simulink model "DPT_model_practice_3"  (R2021b)
settings: Solver=FixedStepAuto  StartTime=0.0  StopTime=0.5  FixedStep=1e-3  RelTol=1e-3
values from neighbouring files (symbols this model uses):
  Jn = 2*Jd    (= 0.000334)    [practice_3_script.m]
  Kd = place(SYS.A,SYS.B,p)    [practice_3_script.m]
  ke = (Un-R*In)/wn    (= 0.320333333333)    [practice_3_script.m]
  km = Mn/In    (= 0.228971962617)    [practice_3_script.m]
  ku = 20    [practice_3_script.m]
  L = l'    [practice_3_script.m]
  La = 10^-3 * 58    (= 0.058)    [practice_3_script.m]
  R = 8.5    [practice_3_script.m]
  SYS = ss(Ad,Bd,Cd,Dd)    [practice_3_script.m]
settings Model: Creator=vkad  LastModifiedBy=vkad

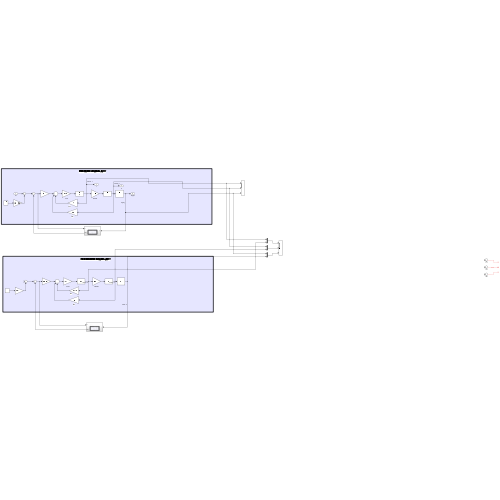
[thumbnail: Simulink's stored preview of the top-level diagram]
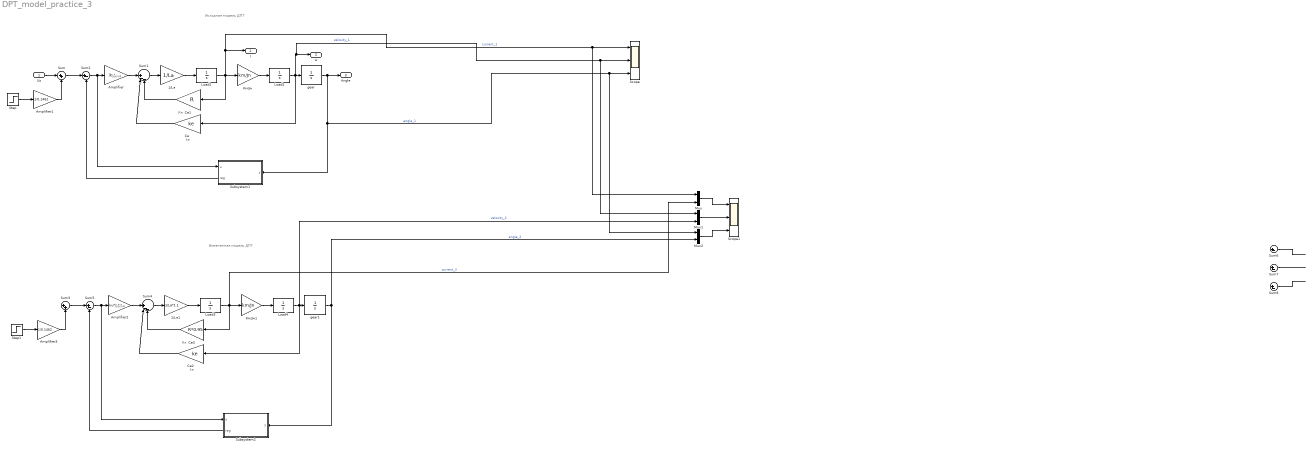
== system DPT_model_practice_3 ==
  note: Rя
  note: Исходная модель ДПТ
  note: Gain4
  note: kе
  note: Rя
  note: Измененная модель ДПТ
  note: Gain4
  note: kе
  Uz : Inport
  1/Lя : Gain  Gain=1/La
  1/Lя1 : Gain  Gain=1/La*1.1
  Amplifier : Gain  Gain=ku
  Amplifier1 : Gain  Gain=1/0.1462
  Amplifier2 : Gain  Gain=ku*0.95
  Amplifier3 : Gain  Gain=1/0.1462
  Ce : Gain  Gain=ke
  Ce1 : Gain  Gain=R
  Ce2 : Gain  Gain=ke
  Ce3 : Gain  Gain=R*0.95
  Load{1..4} (4 alike) : TransferFcn  Denominator=[1 0]
  Mux : Mux  Inputs=2
  Mux1 : Mux  Inputs=2
  Mux2 : Mux  Inputs=2
  Scope : Scope  NumInputPorts=3
  Scope1 : Scope  NumInputPorts=3
  Step : Step  Time=0  SampleTime=0
  Step1 : Step  Time=0  SampleTime=0
  Subsystem1 : Subsystem
      settings: PortSchema="{\"entries\":[{\"content\":{\"sides\":[{\"content\":{\"connectorIds\":[\"In1\",\"Out1\"]},\"type\":\"ConnectorPlacement.EquallySpacedRectSide\",\"uuid\":\"1ae5a343-437d-4cb9-9822-e2db9fa7010c\"},{\"content\":{\"connectorIds\":[\"In2\"],\"side\":\"RIGHT\"},\"type\":\"ConnectorPlacement.EquallySpacedRectSide\",\"uuid\":\"a13fd255-885b-49a4-bdfe-42517e7d2bb6\"},{\"content\":{\"connectorIds\":[],\"side\":\"TOP\"},\"type\":\"ConnectorPlacement.EquallySpacedRectSide\",\"uuid\":\"ec77d7e4-a70f-42b2-8285-e16af54c9a8e\"}]},\"type\":\"ConnectorPlacement.EquallySpacedConnector\",\"uuid\":\"a53451af-0313-4fad-91e1-dbe8374f8c5a\"}],\"packageUris\":[\"http://schema.mathworks.com/mf0/Connector/R2020b\"],\"version\":\"1.0\"}"
  Subsystem2 : Subsystem
      settings: PortSchema="{\"entries\":[{\"content\":{\"sides\":[{\"content\":{\"connectorIds\":[\"In1\",\"Out1\"]},\"type\":\"ConnectorPlacement.EquallySpacedRectSide\",\"uuid\":\"1ae5a343-437d-4cb9-9822-e2db9fa7010c\"},{\"content\":{\"connectorIds\":[\"In2\"],\"side\":\"RIGHT\"},\"type\":\"ConnectorPlacement.EquallySpacedRectSide\",\"uuid\":\"a13fd255-885b-49a4-bdfe-42517e7d2bb6\"},{\"content\":{\"connectorIds\":[],\"side\":\"TOP\"},\"type\":\"ConnectorPlacement.EquallySpacedRectSide\",\"uuid\":\"ec77d7e4-a70f-42b2-8285-e16af54c9a8e\"}]},\"type\":\"ConnectorPlacement.EquallySpacedConnector\",\"uuid\":\"a53451af-0313-4fad-91e1-dbe8374f8c5a\"}],\"packageUris\":[\"http://schema.mathworks.com/mf0/Connector/R2020b\"],\"version\":\"1.0\"}"
  Sum : Sum  Inputs=|++
  Sum1 : Sum  Inputs=||+--
  Sum{2,5..8} (5 alike) : Sum  Inputs=|+-
  Sum3 : Sum  Inputs=|++
  Sum4 : Sum  Inputs=||+--
  gear : TransferFcn  Numerator=1  Denominator=[1 0]
  gear1 : TransferFcn  Numerator=1  Denominator=[1 0]
  Км/Jн : Gain  Gain=km/Jn
  Км/Jн1 : Gain  Gain=km/Jn
  I : Outport
  w : Outport  Port=2
  Angle : Outport  Port=3
  wires:
  Км/Jн/1 -> Load2/1
  Ce/1 -> Sum1/2
  Sum/1 -> Sum2/1
  1/Lя/1 -> Load1/1
  Sum2/1 -> Subsystem1/1(u), Amplifier/1
  Uz/1 -> Sum/1
  Ce1/1 -> Sum1/3
  gear/1 -> Subsystem1/2(y), Mux2/1, Scope/3, Angle/1  "angle_1"
  Step/1 -> Amplifier1/1
  Amplifier/1 -> Sum1/1
  Sum1/1 -> 1/Lя/1
  Load2/1 -> Mux1/1, Scope/2, w/1, Ce/1, gear/1  "velosity_1"
  Load1/1 -> Ce1/1, Км/Jн/1, Mux/1, Scope/1, I/1  "current_1"
  Amplifier1/1 -> Sum/2
  Amplifier3/1 -> Sum3/2
  Subsystem2/1(reg) -> Sum5/2
  Load3/1 -> Mux/2, Км/Jн1/1, Ce3/1  "current_2"
  Load4/1 -> Mux1/2, gear1/1, Ce2/1  "velosity_2"
  Sum4/1 -> 1/Lя1/1
  Amplifier2/1 -> Sum4/1
  Step1/1 -> Amplifier3/1
  gear1/1 -> Mux2/2, Subsystem2/2(y)  "angle_2"
  Ce3/1 -> Sum4/3
  Sum5/1 -> Subsystem2/1(u), Amplifier2/1
  1/Lя1/1 -> Load3/1
  Sum3/1 -> Sum5/1
  Ce2/1 -> Sum4/2
  Км/Jн1/1 -> Load4/1
  Subsystem1/1(reg) -> Sum2/2
  Mux1/1 -> Scope1/2
  Mux2/1 -> Scope1/3
  Mux/1 -> Scope1/1
  Sum8/1 -> ?
  Sum7/1 -> ?
  Sum6/1 -> ?

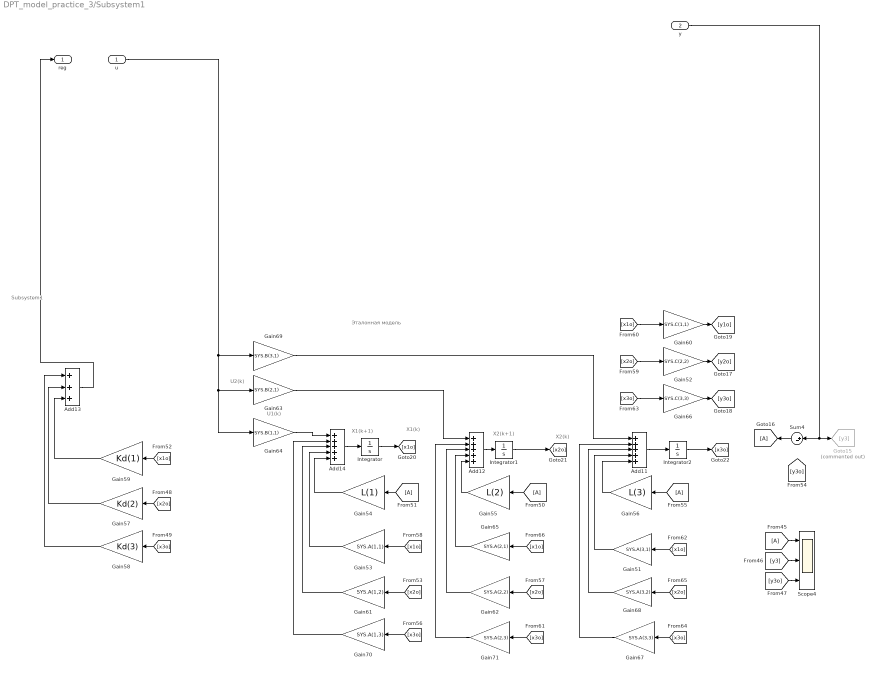
== system DPT_model_practice_3/Subsystem1 ==
  note: Subsystem1
  note: U2(k)
  note: U1(k)
  note: X2(k+1)
  note: X1(k+1)
  note: X2(k)
  note: X1(k)
  note: Эталонная модель
  u : Inport
  y : Inport  Port=2
  Add11 : Sum  Inputs=+++++
  Add12 : Sum  Inputs=+++++
  Add13 : Sum  Inputs=+++
  Add14 : Sum  Inputs=+++++
  Gain51 : Gain  Gain=SYS.A(3,1)
  Gain52 : Gain  Gain=SYS.C(2,2)
  Gain53 : Gain  Gain=SYS.A(1,1)
  Gain54 : Gain  Gain=L(1)
  Gain55 : Gain  Gain=L(2)
  Gain56 : Gain  Gain=L(3)
  Gain57 : Gain  Gain=Kd(2)
  Gain58 : Gain  Gain=Kd(3)
  Gain59 : Gain  Gain=Kd(1)
  Gain60 : Gain  Gain=SYS.C(1,1)
  Gain61 : Gain  Gain=SYS.A(1,2)
  Gain62 : Gain  Gain=SYS.A(2,2)
  Gain63 : Gain  Gain=SYS.B(2,1)
  Gain64 : Gain  Gain=SYS.B(1,1)
  Gain65 : Gain  Gain=SYS.A(2,1)
  Gain66 : Gain  Gain=SYS.C(3,3)
  Gain67 : Gain  Gain=SYS.A(3,3)
  Gain68 : Gain  Gain=SYS.A(3,2)
  Gain69 : Gain  Gain=SYS.B(3,1)
  Gain70 : Gain  Gain=SYS.A(1,3)
  Gain71 : Gain  Gain=SYS.A(2,3)
  Goto15 : Goto  Commented=on  GotoTag=y3
  Integrator : Integrator
  Integrator1 : Integrator
  Integrator2 : Integrator
  Scope4 : Scope  NumInputPorts=3
  Sum4 : Sum  Inputs=|+-
  reg : Outport
  wires:
  u/1 -> Gain69/1, Gain64/1, Gain63/1
  [x1o] -> Gain65/1
  Gain53/1 -> Add14/4
  [y3] -> Scope4/2
  Gain69/1 -> Add11/1
  [A] -> Scope4/1
  [x2o] -> Gain68/1
  Gain61/1 -> Add14/3
  Gain63/1 -> Add12/1
  Gain60/1 -> [y1o]
  [y3o] -> Scope4/3
  [x3o] -> Gain70/1
  [x2o] -> Gain61/1
  Gain58/1 -> Add13/1
  Gain67/1 -> Add11/2
  [A] -> Gain55/1
  Gain54/1 -> Add14/5
  Sum4/1 -> [A]
  y/1 -> Sum4/1, Goto15/1
  [x1o] -> Gain51/1
  Gain59/1 -> Add13/3
  [x3o] -> Gain67/1
  [x1o] -> Gain59/1
  Gain70/1 -> Add14/2
  Gain55/1 -> Add12/5
  [x2o] -> Gain62/1
  [x2o] -> Gain57/1
  [x1o] -> Gain53/1
  [A] -> Gain56/1
  [x1o] -> Gain60/1
  Gain51/1 -> Add11/4
  Gain52/1 -> [y2o]
  Gain71/1 -> Add12/2
  [A] -> Gain54/1
  [x2o] -> Gain52/1
  Gain56/1 -> Add11/5
  Gain62/1 -> Add12/3
  Gain68/1 -> Add11/3
  [x3o] -> Gain71/1
  [x3o] -> Gain58/1
  Gain66/1 -> [y3o]
  Gain64/1 -> Add14/1
  Gain65/1 -> Add12/4
  Gain57/1 -> Add13/2
  [x3o] -> Gain66/1
  Add13/1 -> reg/1
  Add14/1 -> Integrator/1
  Integrator/1 -> [x1o]
  Add12/1 -> Integrator1/1
  Integrator1/1 -> [x2o]
  Add11/1 -> Integrator2/1
  Integrator2/1 -> [x3o]

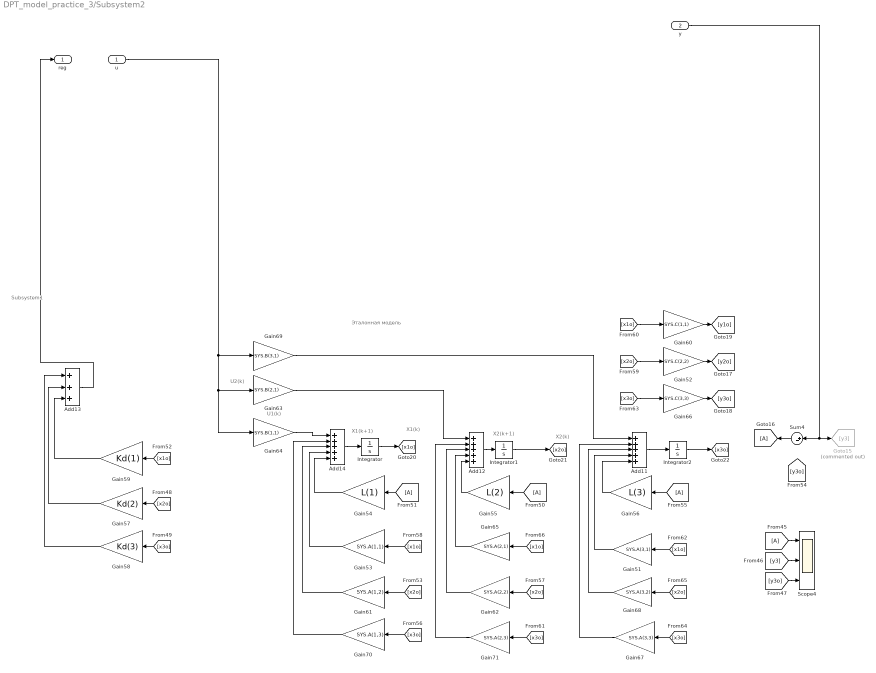
== system DPT_model_practice_3/Subsystem2 ==
  note: Эталонная модель
  note: X1(k)
  note: X2(k)
  note: X1(k+1)
  note: X2(k+1)
  note: U1(k)
  note: U2(k)
  note: Subsystem1
  u : Inport
  y : Inport  Port=2
  Add11 : Sum  Inputs=+++++
  Add12 : Sum  Inputs=+++++
  Add13 : Sum  Inputs=+++
  Add14 : Sum  Inputs=+++++
  Gain51 : Gain  Gain=SYS.A(3,1)
  Gain52 : Gain  Gain=SYS.C(2,2)
  Gain53 : Gain  Gain=SYS.A(1,1)
  Gain54 : Gain  Gain=L(1)
  Gain55 : Gain  Gain=L(2)
  Gain56 : Gain  Gain=L(3)
  Gain57 : Gain  Gain=Kd(2)
  Gain58 : Gain  Gain=Kd(3)
  Gain59 : Gain  Gain=Kd(1)
  Gain60 : Gain  Gain=SYS.C(1,1)
  Gain61 : Gain  Gain=SYS.A(1,2)
  Gain62 : Gain  Gain=SYS.A(2,2)
  Gain63 : Gain  Gain=SYS.B(2,1)
  Gain64 : Gain  Gain=SYS.B(1,1)
  Gain65 : Gain  Gain=SYS.A(2,1)
  Gain66 : Gain  Gain=SYS.C(3,3)
  Gain67 : Gain  Gain=SYS.A(3,3)
  Gain68 : Gain  Gain=SYS.A(3,2)
  Gain69 : Gain  Gain=SYS.B(3,1)
  Gain70 : Gain  Gain=SYS.A(1,3)
  Gain71 : Gain  Gain=SYS.A(2,3)
  Goto15 : Goto  Commented=on  GotoTag=y3
  Integrator : Integrator
  Integrator1 : Integrator
  Integrator2 : Integrator
  Scope4 : Scope  NumInputPorts=3
  Sum4 : Sum  Inputs=|+-
  reg : Outport
  wires:
  Integrator2/1 -> [x3o]
  Add11/1 -> Integrator2/1
  Integrator1/1 -> [x2o]
  Add12/1 -> Integrator1/1
  Integrator/1 -> [x1o]
  Add14/1 -> Integrator/1
  Add13/1 -> reg/1
  [x3o] -> Gain66/1
  Gain57/1 -> Add13/2
  Gain65/1 -> Add12/4
  Gain64/1 -> Add14/1
  Gain66/1 -> [y3o]
  [x3o] -> Gain58/1
  [x3o] -> Gain71/1
  Gain68/1 -> Add11/3
  Gain62/1 -> Add12/3
  Gain56/1 -> Add11/5
  [x2o] -> Gain52/1
  [A] -> Gain54/1
  Gain71/1 -> Add12/2
  Gain52/1 -> [y2o]
  Gain51/1 -> Add11/4
  [x1o] -> Gain60/1
  [A] -> Gain56/1
  [x1o] -> Gain53/1
  [x2o] -> Gain57/1
  [x2o] -> Gain62/1
  Gain55/1 -> Add12/5
  Gain70/1 -> Add14/2
  [x1o] -> Gain59/1
  [x3o] -> Gain67/1
  Gain59/1 -> Add13/3
  [x1o] -> Gain51/1
  y/1 -> Goto15/1, Sum4/1
  Sum4/1 -> [A]
  Gain54/1 -> Add14/5
  [A] -> Gain55/1
  Gain67/1 -> Add11/2
  Gain58/1 -> Add13/1
  [x2o] -> Gain61/1
  [x3o] -> Gain70/1
  [y3o] -> Scope4/3
  Gain60/1 -> [y1o]
  Gain63/1 -> Add12/1
  Gain61/1 -> Add14/3
  [x2o] -> Gain68/1
  [A] -> Scope4/1
  Gain69/1 -> Add11/1
  [y3] -> Scope4/2
  Gain53/1 -> Add14/4
  [x1o] -> Gain65/1
  u/1 -> Gain63/1, Gain64/1, Gain69/1
